simulink model "Control_Planta_LazoCerrado"  (R2023b)
settings: Solver=VariableStepAuto  StartTime=0.0  StopTime=15  FixedStep=0.00001  RelTol=1e-3
values from neighbouring files (symbols this model uses):
  A_corriente = [0 1; -wn_corriente^2 -2*zeta_corriente*wn_corriente]    [SensoresReales.m]
  A_inv = [0 1; -wn_inv^2 -2*zeta_inv*wn_inv]    [SensoresReales.m]
  A_temp = -1/tau_temp    (= -0.05)    [SensoresReales.m]
  A_tita = [0 1; -wn_tita^2 -2*zeta_tita*wn_tita]    [SensoresReales.m]
  B_corriente = [0; wn_corriente^2]    [SensoresReales.m]
  B_inv = [0; wn_inv^2]    [SensoresReales.m]
  B_temp = 1/tau_temp    (= 0.05)    [SensoresReales.m]
  B_tita = [0; wn_tita^2]    [SensoresReales.m]
  C_corriente = [1 0]    [SensoresReales.m]
  C_inv = [1 0]    [SensoresReales.m]
  C_temp = 1    [SensoresReales.m]
  C_tita = [1 0]    [SensoresReales.m]
  D_corriente = 0    [SensoresReales.m]
  D_inv = 0    [SensoresReales.m]
  D_temp = 0    [SensoresReales.m]
  D_tita = 0    [SensoresReales.m]
  id_consigna = 0.5    [RdLazoCorriente.m]
  ketita = double(sol.ketita_s)    [PIDPolosObsReducidoEst.m]    (also in PolosObsReducidoEst.m)
  kew = double(sol.kew_s)    [PIDPolosObsReducidoEst.m]    (also in PolosObsReducidoEst.m)
  kewint = double(sol.kewint_s)    [PIDPolosObsReducidoEst.m]    (also in PolosObsReducidoEst.m = 0)
  Ra_prima = Lq/Tau    [RaLazoControlCorriente.m]
  Rd_prima = Ld/Tau_d    [RdLazoCorriente.m]
  Tau = -1/Pi    (= 0.0002)    [RaLazoControlCorriente.m]
  Ts = 0.0001    [TustinPID.m]
  Vs_max = 48 * sqrt(2) / sqrt(3)    [SensoresReales.m]
undefined symbols (not defined in the file or in its folder): alfa, beq, Cts, den_PIDTZ, DiscIntNeverNeededParam, g, id0, io0, iq0, Ismax, Isnom, Jeq, KEeq, kl, KTeq, lambda_m, Ld, Lls, Lq, num_PIDTZ, Pp, r, Rs, Rts_amb, tita0, Tqnom, Ts0, Tsmax, Vflnom, Wlnom, wm0, Wmnom
libraries: simulink x11, simulink_extras x8, eeTransforms x4, SignalEditorBlockLib x3, dspsigops x1, spsabctoAlphaBetaZeroLib x1
settings Model: Creator=Julian  LastModifiedBy=Gustavo

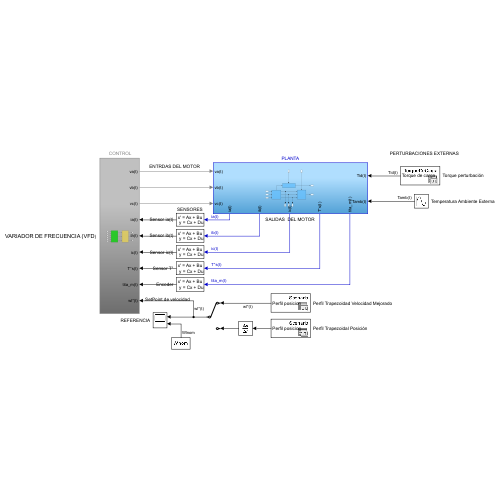
[thumbnail: Simulink's stored preview of the top-level diagram]
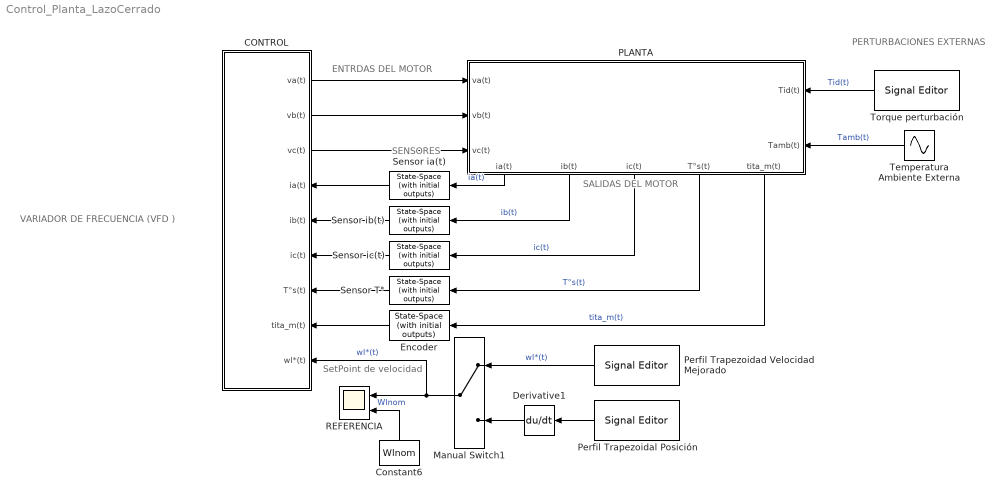
== system Control_Planta_LazoCerrado ==
  note: VARIADOR DE FRECUENCIA (VFD )
  note: SENSORES
  note: ENTRDAS DEL MOTOR
  note: PERTURBACIONES EXTERNAS
  note: SetPoint de velocidad
  note: SALIDAS DEL MOTOR
  " CONTROL" : Subsystem
      settings: PortSchema="{\"entries\":[{\"content\":{\"sides\":[{\"content\":{},\"type\":\"ConnectorPlacement.EquallySpacedRectSide\",\"uuid\":\"d9793d3b-98b9-44dc-9764-d251b8ee8eaa\"},{\"content\":{\"connectorIds\":[\"Out1\",\"Out2\",\"Out3\",\"In1\",\"In2\",\"In3\",\"In4\",\"In5\",\"In6\"],\"side\":\"RIGHT\"},\"type\":\"ConnectorPlacement.EquallySpacedRectSide\",\"uuid\":\"bdddef0b-c469-49f9-98ba-074ea9cbca1a\"},{\"content\":{\"side\":\"TOP\"},\"type\":\"ConnectorPlacement.EquallySpacedRectSide\",\"uuid\":\"8ca6b3a1-550b-497a-8309-d6b694c418e8\"}]},\"type\":\"ConnectorPlacement.EquallySpacedConnector\",\"uuid\":\"d8d4494b-c45d-4f5a-9083-73b1f67c784a\"}],\"packageUris\":[\"http://schema.mathworks.com/mf0/Connector/R2020b\"],\"version\":\"1.0\"}"
  Constant6 : Constant  Value=Wlnom
  Derivative1 : Derivative
  Encoder : simulink_extras/Additional Linear/State-Space (with initial outputs)  A=A_tita  B=B_tita  C=C_tita  D=D_tita  U0=0  Y0=0
  Manual Switch1 : ManualSwitch
  PLANTA : Subsystem
      settings: PortSchema="{\"entries\":[{\"content\":{\"sides\":[{\"content\":{\"connectorIds\":[\"In1\",\"In2\",\"In3\"]},\"type\":\"ConnectorPlacement.EquallySpacedRectSide\",\"uuid\":\"c9ff8e03-575d-49b6-9d53-263c6173ec7a\"},{\"content\":{\"connectorIds\":[\"In4\",\"In5\"],\"side\":\"RIGHT\"},\"type\":\"ConnectorPlacement.EquallySpacedRectSide\",\"uuid\":\"b812656a-111e-4032-91bd-eba1e3276cdf\"},{\"content\":{\"side\":\"TOP\"},\"type\":\"ConnectorPlacement.EquallySpacedRectSide\",\"uuid\":\"1a03caaa-7f6e-4ad3-ab54-ee47607f786a\"},{\"content\":{\"connectorIds\":[\"Out1\",\"Out2\",\"Out3\",\"Out4\",\"Out5\"],\"side\":\"BOTTOM\"},\"type\":\"ConnectorPlacement.EquallySpacedRectSide\",\"uuid\":\"9d23a867-d392-4f38-a76b-2655c4618fc4\"}]},\"type\":\"ConnectorPlacement.EquallySpacedConnector\",\"uuid\":\"9323b1ce-1fa4-461e-b8aa-3e94b35b1dab\"}],\"packageUris\":[\"http://schema.mathworks.com/mf0/Connector/R2020b\"],\"version\":\"1.0\"}"
  Perfil Trapezoidad Velocidad Mejorado : SignalEditorBlockLib/Signal Editor  FileName=PerfilTrapezoidalVelocidadMejorado.mat  ActiveScenario=Scenario  ActiveSignal=Perfil posicion  IsBus=off  OutputBusObjectStr=Bus: BusObject  SampleTime=0  ZeroCross=off  OutputAfterFinalValue=Setting to zero  Unit=inherit  PreserveSignalName=on  ApplySigPropsToAllScenarios=on  ApplySigPropsToAllSignals=off
  Perfil Trapezoidal Posición : SignalEditorBlockLib/Signal Editor  FileName=Perfil trapezoidal de posicion.mat  ActiveScenario=Scenario  ActiveSignal=Perfil posicion  IsBus=off  OutputBusObjectStr=Bus: BusObject  SampleTime=0  ZeroCross=off  OutputAfterFinalValue=Setting to zero  Unit=inherit  PreserveSignalName=on  ApplySigPropsToAllScenarios=on  ApplySigPropsToAllSignals=off
  REFERENCIA : Scope  NumInputPorts=2
  Sensor T° : simulink_extras/Additional Linear/State-Space (with initial outputs)  A=A_temp  B=B_temp  C=C_temp  D=D_temp  U0=40  Y0=40
  Sensor ia(t) : simulink_extras/Additional Linear/State-Space (with initial outputs)  A=A_corriente  B=B_corriente  C=C_corriente  D=D_corriente  U0=0  Y0=0
  Sensor ib(t) : simulink_extras/Additional Linear/State-Space (with initial outputs)  A=A_corriente  B=B_corriente  C=C_corriente  D=D_corriente  U0=0  Y0=0
  Sensor ic(t) : simulink_extras/Additional Linear/State-Space (with initial outputs)  A=A_corriente  B=B_corriente  C=C_corriente  D=D_corriente  U0=0  Y0=0
  Temperatura Ambiente Externa : Sin  Amplitude=27.5  Bias=12.5  Frequency=2*pi/15  Phase=pi/2  SampleTime=0
  Torque perturbación : SignalEditorBlockLib/Signal Editor  FileName=Torque de carga Tdl(t).mat  ActiveScenario=TorqueDeCarga  ActiveSignal=Torque de carga  IsBus=off  OutputBusObjectStr=Bus: BusObject  SampleTime=0  ZeroCross=off  OutputAfterFinalValue=Setting to zero  Unit=N*m  PreserveSignalName=on  ApplySigPropsToAllScenarios=on  ApplySigPropsToAllSignals=off
  wires:
  Torque perturbación/1 -> PLANTA/4(Tid(t))  "Tid(t)"
  PLANTA/5(tita_m(t)) -> Encoder/1  "tita_m(t)"
  PLANTA/1(ia(t)) -> Sensor ia(t)/1  "ia(t)"
  Manual Switch1/1 -> " CONTROL"/6(wl*(t)), REFERENCIA/1  "wl*(t)"
  Perfil Trapezoidad Velocidad Mejorado/1 -> Manual Switch1/1  "wl*(t)"
  Perfil Trapezoidal Posición/1 -> Derivative1/1
  Derivative1/1 -> Manual Switch1/2
  Constant6/1 -> REFERENCIA/2  "Wlnom"
  Temperatura Ambiente Externa/1 -> PLANTA/5(Tamb(t))  "Tamb(t)"
  PLANTA/4(T°s(t)) -> Sensor T°/1  "T°s(t)"
  PLANTA/2(ib(t)) -> Sensor ib(t)/1  "ib(t)"
  " CONTROL"/1(va(t)) -> PLANTA/1(va(t))
  " CONTROL"/2(vb(t)) -> PLANTA/2(vb(t))
  " CONTROL"/3(vc(t)) -> PLANTA/3(vc(t))
  Sensor ia(t)/1 -> " CONTROL"/1(ia(t))
  Sensor ib(t)/1 -> " CONTROL"/2(ib(t))
  Sensor ic(t)/1 -> " CONTROL"/3(ic(t))
  PLANTA/3(ic(t)) -> Sensor ic(t)/1  "ic(t)"
  Encoder/1 -> " CONTROL"/5(tita_m(t))
  Sensor T°/1 -> " CONTROL"/4(T°s(t))

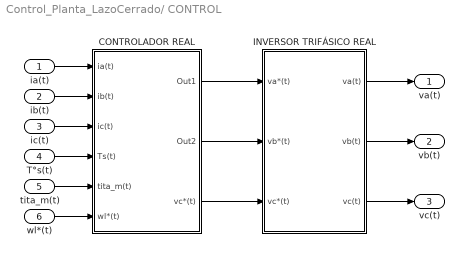
== system Control_Planta_LazoCerrado/ CONTROL ==
  ia(t) : Inport
  ib(t) : Inport  Port=2
  ic(t) : Inport  Port=3
  T°s(t) : Inport  Port=4
  tita_m(t) : Inport  Port=5
  wl*(t) : Inport  Port=6
  CONTROLADOR REAL : Subsystem
  INVERSOR TRIFÁSICO REAL : Subsystem
  va(t) : Outport
  vb(t) : Outport  Port=2
  vc(t) : Outport  Port=3
  wires:
  T°s(t)/1 -> CONTROLADOR REAL/4(Ts(t))
  CONTROLADOR REAL/2(Out2) -> INVERSOR TRIFÁSICO REAL/2(vb*(t))
  CONTROLADOR REAL/1(Out1) -> INVERSOR TRIFÁSICO REAL/1(va*(t))
  wl*(t)/1 -> CONTROLADOR REAL/6(wl*(t))
  INVERSOR TRIFÁSICO REAL/2(vb(t)) -> vb(t)/1
  ib(t)/1 -> CONTROLADOR REAL/2(ib(t))
  CONTROLADOR REAL/3(vc*(t)) -> INVERSOR TRIFÁSICO REAL/3(vc*(t))
  ia(t)/1 -> CONTROLADOR REAL/1(ia(t))
  ic(t)/1 -> CONTROLADOR REAL/3(ic(t))
  INVERSOR TRIFÁSICO REAL/1(va(t)) -> va(t)/1
  INVERSOR TRIFÁSICO REAL/3(vc(t)) -> vc(t)/1
  tita_m(t)/1 -> CONTROLADOR REAL/5(tita_m(t))

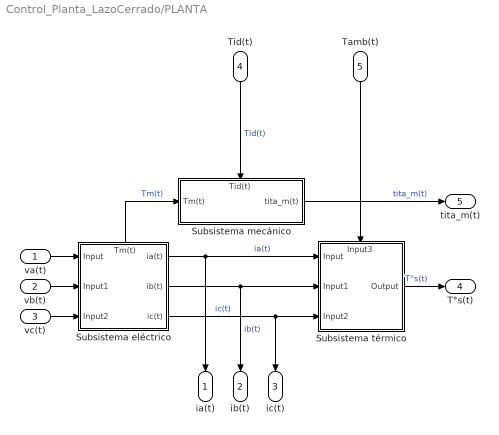
== system Control_Planta_LazoCerrado/PLANTA ==
  va(t) : Inport
  vb(t) : Inport  Port=2
  vc(t) : Inport  Port=3
  Tid(t) : Inport  Port=4
  Tamb(t) : Inport  Port=5
  Subsistema eléctrico : Subsystem
      settings: PortSchema="{\"entries\":[{\"content\":{\"sides\":[{\"content\":{\"connectorIds\":[\"In1\",\"In2\",\"In3\"]},\"type\":\"ConnectorPlacement.EquallySpacedRectSide\",\"uuid\":\"55314de5-b6ab-4161-b15d-819ac9b3d610\"},{\"content\":{\"connectorIds\":[\"Out1\",\"Out2\",\"Out3\"],\"side\":\"RIGHT\"},\"type\":\"ConnectorPlacement.EquallySpacedRectSide\",\"uuid\":\"6d89c228-26ff-4db5-b942-5bfef0be2fde\"},{\"content\":{\"connectorIds\":[\"Out4\"],\"side\":\"TOP\"},\"type\":\"ConnectorPlacement.EquallySpacedRectSide\",\"uuid\":\"a52f3ca3-a7f6-4886-b92b-9c9e6a107711\"}]},\"type\":\"ConnectorPlacement.EquallySpacedConnector\",\"uuid\":\"22991da4-d60d-4ddc-8bfe-b68e23663f11\"}],\"packageUris\":[\"http://schema.mathworks.com/mf0/Connector/R2020b\"],\"version\":\"1.0\"}"
  Subsistema mecánico : Subsystem
      settings: PortSchema="{\"entries\":[{\"content\":{\"sides\":[{\"content\":{\"connectorIds\":[\"In1\"]},\"type\":\"ConnectorPlacement.EquallySpacedRectSide\",\"uuid\":\"db0c31ff-fb9a-4cce-bd75-6b297d65744d\"},{\"content\":{\"connectorIds\":[\"Out1\"],\"side\":\"RIGHT\"},\"type\":\"ConnectorPlacement.EquallySpacedRectSide\",\"uuid\":\"ab44173d-bb84-4ea2-b7b7-ef15b1ff9d5e\"},{\"content\":{\"connectorIds\":[\"In2\"],\"side\":\"TOP\"},\"type\":\"ConnectorPlacement.EquallySpacedRectSide\",\"uuid\":\"a2ba5669-abba-4e87-b14b-37ec0d904023\"}]},\"type\":\"ConnectorPlacement.EquallySpacedConnector\",\"uuid\":\"7722c9ef-afaa-4930-9e2a-97c0dfb446ab\"}],\"packageUris\":[\"http://schema.mathworks.com/mf0/Connector/R2020b\"],\"version\":\"1.0\"}"
  Subsistema térmico : Subsystem
      settings: PortSchema="{\"entries\":[{\"content\":{\"sides\":[{\"content\":{\"connectorIds\":[\"In1\",\"In2\",\"In3\"]},\"type\":\"ConnectorPlacement.EquallySpacedRectSide\",\"uuid\":\"499bb5e3-da94-498d-be5e-1974ba0b4a58\"},{\"content\":{\"connectorIds\":[\"Out1\"],\"side\":\"RIGHT\"},\"type\":\"ConnectorPlacement.EquallySpacedRectSide\",\"uuid\":\"13ea5dea-e51e-4770-b579-88e3e6e50884\"},{\"content\":{\"connectorIds\":[\"In4\"],\"side\":\"TOP\"},\"type\":\"ConnectorPlacement.EquallySpacedRectSide\",\"uuid\":\"72517ed1-a98f-428e-86e2-c370e237c602\"}]},\"type\":\"ConnectorPlacement.EquallySpacedConnector\",\"uuid\":\"7e0eda24-12d6-49d0-ad1f-024c88e78140\"}],\"packageUris\":[\"http://schema.mathworks.com/mf0/Connector/R2020b\"],\"version\":\"1.0\"}"
  ia(t) : Outport
  ib(t) : Outport  Port=2
  ic(t) : Outport  Port=3
  T°s(t) : Outport  Port=4
  tita_m(t) : Outport  Port=5
  wires:
  Tamb(t)/1 -> Subsistema térmico/4(Input3)
  Subsistema eléctrico/3(ic(t)) -> Subsistema térmico/3(Input2), ic(t)/1  "ic(t)"
  Subsistema eléctrico/1(ia(t)) -> Subsistema térmico/1(Input), ia(t)/1  "ia(t)"
  Subsistema térmico/1(Output) -> T°s(t)/1  "T°s(t)"
  Subsistema eléctrico/4(Tm(t)) -> Subsistema mecánico/1(Tm(t))  "Tm(t)"
  Subsistema eléctrico/2(ib(t)) -> Subsistema térmico/2(Input1), ib(t)/1  "ib(t)"
  Subsistema mecánico/1(tita_m(t)) -> tita_m(t)/1  "tita_m(t)"
  va(t)/1 -> Subsistema eléctrico/1(Input)
  vb(t)/1 -> Subsistema eléctrico/2(Input1)
  Tid(t)/1 -> Subsistema mecánico/2(Tid(t))  "Tid(t)"
  vc(t)/1 -> Subsistema eléctrico/3(Input2)

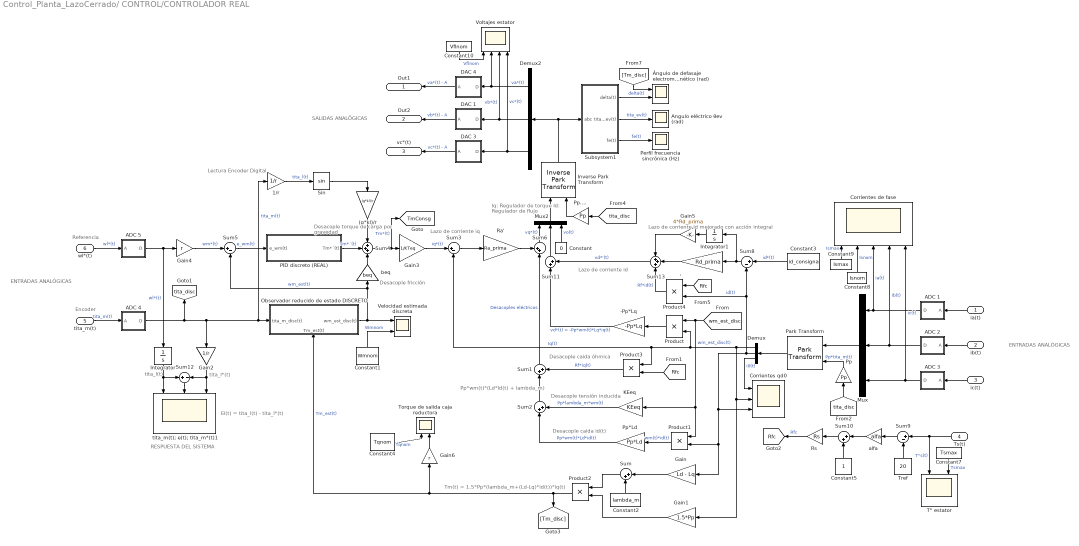
== system Control_Planta_LazoCerrado/ CONTROL/CONTROLADOR REAL ==
  note: Lazo de corriente id mejorado con acción integral
  note: Iq: Regulador de torque
      | Id: Regulador de flujo
  note: Lazo de corriente id
  note: ENTRADAS ANALÓGICAS
  note: SALIDAS ANALÖGICAS
  note: Desacople caida id(t)
  note: Encoder
  note: Desacople caida óhmica
  note: Desacople fricción
  note: Desacople tensión inducida
  note: Pp*wm(t)*(Ld*Id(t) + lambda_m)
  note: Lectura Encoder Digital
  note: Desacople torque
      | de carga por gravedad
  note: Tm(t) = 1.5*Pp*(lambda_m+(Ld-Lq)*id(t))*iq(t)
  note: ENTRADAS ANALÓGICAS
  note: Referencia
  note: Lazo de corriente iq
  note: tita_l*(t)
  note: RESPUESTA DEL SISTEMA
  note: El(t) = tita_l(t) - tita_l*(t)
  note: tita_l(t)
  ia(t) : Inport
  ib(t) : Inport  Port=2
  ic(t) : Inport  Port=3
  Ts(t) : Inport  Port=4
  tita_m(t) : Inport  Port=5
  wl*(t) : Inport  Port=6
  ' : Gain  Gain=Rd_prima
  (g*kl)/r : Gain  Gain=(g*kl)/r
  -Pp*Lq : Gain  Gain=-Pp*Lq
  1/r : Gain  Gain=1/r
  ADC 1 : Subsystem
  ADC 2 : Subsystem
  ADC 3 : Subsystem
  ADC 4 : Subsystem
  ADC 5 : Subsystem
  Angulo eléctrico θev (rad) : Scope
  Constant : Constant  Value=0
  Constant1 : Constant  Value=Wmnom
  Constant10 : Constant  Value=Vflnom
  Constant2 : Constant  Value=lambda_m
  Constant3 : Constant  Value=id_consigna
  Constant4 : Constant  Value=Tqnom
  Constant5 : Constant
  Constant7 : Constant  Value=Tsmax
  Constant8 : Constant  Value=Isnom
  Constant9 : Constant  Value=Ismax
  Corrientes de fase : Scope  NumInputPorts=5
  Corrientes qd0 : Scope  NumInputPorts=3
  DAC 1 : Subsystem
  DAC 3 : Subsystem
  DAC 4 : Subsystem
  Demux : Demux  Outputs=3
  Demux2 : Demux  Outputs=3
  Gain : Gain  Gain=Ld - Lq
  Gain1 : Gain  Gain=1.5*Pp
  Gain2 : Gain  Gain=1/r
  Gain3 : Gain  Gain=1/KTeq
  Gain4 : Gain  Gain=r
  Gain5 : Gain  Gain=4*Rd_prima
  Gain6 : Gain  Gain=r
  Integrator : Integrator
  Integrator1 : Integrator
  Inverse Park Transform : eeTransforms/Inverse Park Transform  AxisAlignment=Q-axis  PowerInvariant=off
      settings: LibrarySourceBlock=|
      | ee_sl_lib/Mathematical
      | Transforms/Inverse
      | Park Transform
  KEeq : Gain  Gain=KEeq
  Mux : Mux  Inputs=3
  Mux2 : Mux  Inputs=3
  Observador reducido de estado DISCRETO : Subsystem
      settings: PortSchema="{\"entries\":[{\"content\":{\"sides\":[{\"content\":{\"connectorIds\":[\"In1\"]},\"type\":\"ConnectorPlacement.EquallySpacedRectSide\",\"uuid\":\"14c71593-68f9-47eb-b449-943d4a083251\"},{\"content\":{\"connectorIds\":[\"Out1\"],\"side\":\"RIGHT\"},\"type\":\"ConnectorPlacement.EquallySpacedRectSide\",\"uuid\":\"16b08435-5727-4596-8f16-f9c2ce0b209d\"},{\"content\":{\"side\":\"TOP\"},\"type\":\"ConnectorPlacement.EquallySpacedRectSide\",\"uuid\":\"cb5316ed-c33b-4267-9a86-77fc386a7eee\"},{\"content\":{\"connectorIds\":[\"In2\"],\"side\":\"BOTTOM\"},\"type\":\"ConnectorPlacement.EquallySpacedRectSide\",\"uuid\":\"5f586da6-a83e-437c-ae41-e23b930b940a\"}]},\"type\":\"ConnectorPlacement.EquallySpacedConnector\",\"uuid\":\"0742f703-5bdc-4b50-9418-7ea0767d1226\"}],\"packageUris\":[\"http://schema.mathworks.com/mf0/Connector/R2020b\"],\"version\":\"1.0\"}"
  PID discreto (REAL) : Subsystem
  Park Transform : eeTransforms/Park Transform  AxisAlignment=Q-axis  PowerInvariant=off
      settings: LibrarySourceBlock=|
      | ee_sl_lib/Mathematical
      | Transforms/Park Transform
  Perfil frecuencia sincrónica (Hz) : Scope
  Pp : Gain  Gain=Pp
  Pp*Ld : Gain  Gain=Pp*Ld
  Pp.... : Gain  Gain=Pp
  Product{,1..4} (5 alike) : Product
  Ra' : Gain  Gain=Ra_prima
  Rs : Gain  Gain=Rs
  Sin : Trigonometry
  Subsystem1 : Subsystem
  Sum{,1..2,10..11} (5 alike) : Sum  Inputs=|++
  Sum12 : Sum  Inputs=+|-
  Sum13 : Sum  Inputs=+++
  Sum{3,5,8..9} (4 alike) : Sum  Inputs=|+-
  Sum4 : Sum  Inputs=+++
  Sum6 : Sum  Inputs=++|
  Torque de salida caja reductora : Scope  NumInputPorts=2
  Tref : Constant  Value=20
  T° estator : Scope  NumInputPorts=2
  Velocidad estimada discreta : Scope  NumInputPorts=2
  Voltajes estator : Scope  NumInputPorts=4
  alfa : Gain  Gain=alfa
  beq : Gain  Gain=beq
  tita_m(t); e(t); tita_m*(t)1 : Scope  NumInputPorts=3
  Ángulo de defasaje electromagnético (rad) : Scope  NumInputPorts=2
  Out1 : Outport
  Out2 : Outport  Port=2
  vc*(t) : Outport  Port=3
  tag scope: Rfc=global, TmConsg=global, tita_disc=global
  wires:
  Mux/1 -> Park Transform/1
  [tita_disc] -> Pp..../1
  Pp..../1 -> Inverse Park Transform/2
  Constant/1 -> Mux2/3  "vo(t)"
  Product3/1 -> Sum1/2  "Rf*iq(t)"
  [tita_disc] -> Pp/1
  Ra'/1 -> Sum6/1
  Inverse Park Transform/1 -> Subsystem1/1(abc), Demux2/1
  KEeq/1 -> Sum2/2  "Pp*lambda_m*wm(t)"
  Product1/1 -> Pp*Ld/1  "wm(t)*id(t)"
  Mux2/1 -> Inverse Park Transform/1
  Sum2/1 -> Sum1/1
  wl*(t)/1 -> ADC 5/1(A)  "wl*(t)"
  Pp*Ld/1 -> Sum2/1  "Pp*wm(t)*Ld*id(t)"
  Gain3/1 -> Sum3/1  "iq*(t)"
  Product/1 -> -Pp*Lq/1
  Park Transform/1 -> Demux/1
  Pp/1 -> Park Transform/2  "Pp*tita_m(t)"
  Sum6/1 -> Mux2/1  "vq*(t)"
  tita_m(t)/1 -> ADC 4/1(A)  "tita_m(t)"
  [Rfc] -> Product3/2
  Sum1/1 -> Sum6/2  "Desacoples eléctricos"
  Sum4/1 -> [TmConsg], Gain3/1  "Tm*(t)"
  beq/1 -> Sum4/3
  Observador reducido de estado DISCRETO/1(wm_est_disc(t)) -> Sum5/2, beq/1, Velocidad estimada discreta/1  "wm_est(t)"
  Demux/3 -> Corrientes qd0/1  "i0(t)"
  Demux/1 -> Product3/1, Sum3/2, Product/2, Gain1/1, Corrientes qd0/2  "Iq(t)"
  1/r/1 -> Sin/1  "tita_l(t)"
  Sin/1 -> (g*kl)/r/1
  (g*kl)/r/1 -> Sum4/1
  [wm_est_disc] -> Product1/1, KEeq/1, Product/1  "wm_est_disc(t)"
  Constant1/1 -> Velocidad estimada discreta/2  "Wmnom"
  ia(t)/1 -> ADC 1/1(A)
  ib(t)/1 -> ADC 2/1(A)
  ic(t)/1 -> ADC 3/1(A)
  ADC 1/1(D) -> Corrientes de fase/3, Mux/1  "ia(t)"
  Sum/1 -> Product2/1
  Constant2/1 -> Sum/2
  Gain1/1 -> Product2/2
  Gain/1 -> Sum/1
  DAC 4/1(A) -> Out1/1  "va*(t) - A"
  DAC 1/1(A) -> Out2/1  "vb*(t) - A"
  DAC 3/1(A) -> vc*(t)/1  "vc*(t) - A"
  Sum3/1 -> Ra'/1
  PID discreto (REAL)/1(Tm*´(t)) -> Sum4/2  "Tm*´(t)"
  Sum5/1 -> PID discreto (REAL)/1(e_wm(t))  "e_wm(t)"
  Subsystem1/2(tita_ev(t)) -> Angulo eléctrico θev (rad)/1  "tita_ev(t)"
  Subsystem1/1(delta(t)) -> Ángulo de defasaje electromagnético (rad)/2  "delta(t)"
  Subsystem1/3(fe(t)) -> Perfil frecuencia sincrónica (Hz)/1  "fe(t)"
  Sum9/1 -> alfa/1
  Sum10/1 -> Rs/1
  Rs/1 -> [Rfc]  "Rfc"
  [Rfc] -> Product4/1
  Product4/1 -> Sum13/3  "Rf*id(t)"
  Constant3/1 -> Sum8/1  "id*(t)"
  Sum8/1 -> Integrator1/1, '/1
  Demux/2 -> Sum8/2, Product4/2, Gain/1, Product1/2, Corrientes qd0/3  "id(t)"
  -Pp*Lq/1 -> Sum11/1  "vd*(t) = -Pp*wm(t)*Lq*iq(t)"
  Sum11/1 -> Mux2/2
  [Tm_disc] -> Ángulo de defasaje electromagnético (rad)/1
  Tref/1 -> Sum9/2
  Constant5/1 -> Sum10/2
  alfa/1 -> Sum10/1
  Demux2/3 -> DAC 3/1(D), Voltajes estator/4  "vc*(t)"
  Demux2/1 -> Voltajes estator/2, DAC 4/1(D)  "va*(t)"
  Demux2/2 -> DAC 1/1(D), Voltajes estator/3  "vb*(t)"
  Constant10/1 -> Voltajes estator/1  "Vflnom"
  Constant9/1 -> Corrientes de fase/1  "Ismax"
  ADC 3/1(D) -> Corrientes de fase/5, Mux/3  "ic(t)"
  ADC 2/1(D) -> Corrientes de fase/4, Mux/2  "ib(t)"
  Constant8/1 -> Corrientes de fase/2  "Isnom"
  Ts(t)/1 -> Sum9/1, T° estator/1  "T°s(t)"
  Constant7/1 -> T° estator/2  "Tsmax"
  ADC 4/1(D) -> Gain2/1, 1/r/1, Observador reducido de estado DISCRETO/1(tita_m_disc(t)), [tita_disc]  "tita_m(t)"
  ADC 5/1(D) -> Gain4/1, Integrator/1  "wl*(t)"
  Sum12/1 -> tita_m(t); e(t); tita_m*(t)1/2
  Gain4/1 -> Sum5/1  "wm*(t)"
  Gain2/1 -> Sum12/2, tita_m(t); e(t); tita_m*(t)1/3
  Integrator/1 -> tita_m(t); e(t); tita_m*(t)1/1, Sum12/1
  Sum13/1 -> Sum11/2  "vd*'(t)"
  Integrator1/1 -> Gain5/1
  Gain5/1 -> Sum13/1
  '/1 -> Sum13/2
  Product2/1 -> [Tm_disc], Gain6/1, Observador reducido de estado DISCRETO/2(Tm_est(t))  "Tm_est(t)"
  Gain6/1 -> Torque de salida caja reductora/2
  Constant4/1 -> Torque de salida caja reductora/1  "Tqnom"

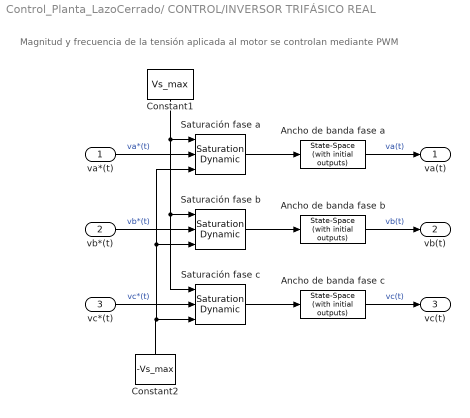
== system Control_Planta_LazoCerrado/ CONTROL/INVERSOR TRIFÁSICO REAL ==
  note: Magnitud y frecuencia de la tensión aplicada al motor se controlan mediante PWM
  va*(t) : Inport
  vb*(t) : Inport  Port=2
  vc*(t) : Inport  Port=3
  Ancho de banda fase a : simulink_extras/Additional Linear/State-Space (with initial outputs)  A=A_inv  B=B_inv  C=C_inv  D=D_inv  U0=0  Y0=0
  Ancho de banda fase b : simulink_extras/Additional Linear/State-Space (with initial outputs)  A=A_inv  B=B_inv  C=C_inv  D=D_inv  U0=0  Y0=0
  Ancho de banda fase c : simulink_extras/Additional Linear/State-Space (with initial outputs)  A=A_inv  B=B_inv  C=C_inv  D=D_inv  U0=0  Y0=0
  Constant1 : Constant  Value=Vs_max
  Constant2 : Constant  Value=-Vs_max
  Saturación fase a : simulink/Discontinuities/Saturation Dynamic  OutMin=[]  OutMax=[]  OutDataTypeStr=Inherit: Same as second input  OutDataType=fixdt(1, 16)  OutScaling=2^-10  DoSatur=off
  Saturación fase b : simulink/Discontinuities/Saturation Dynamic  OutMin=[]  OutMax=[]  OutDataTypeStr=Inherit: Same as second input  OutDataType=fixdt(1, 16)  OutScaling=2^-10  DoSatur=off
  Saturación fase c : simulink/Discontinuities/Saturation Dynamic  OutMin=[]  OutMax=[]  OutDataTypeStr=Inherit: Same as second input  OutDataType=fixdt(1, 16)  OutScaling=2^-10  DoSatur=off
  va(t) : Outport
  vb(t) : Outport  Port=2
  vc(t) : Outport  Port=3
  wires:
  Constant2/1 -> Saturación fase c/3, Saturación fase a/3, Saturación fase b/3
  va*(t)/1 -> Saturación fase a/2  "va*(t)"
  Saturación fase c/1 -> Ancho de banda fase c/1
  vc*(t)/1 -> Saturación fase c/2  "vc*(t)"
  vb*(t)/1 -> Saturación fase b/2  "vb*(t)"
  Saturación fase b/1 -> Ancho de banda fase b/1
  Saturación fase a/1 -> Ancho de banda fase a/1
  Constant1/1 -> Saturación fase c/1, Saturación fase b/1, Saturación fase a/1
  Ancho de banda fase b/1 -> vb(t)/1  "vb(t)"
  Ancho de banda fase a/1 -> va(t)/1  "va(t)"
  Ancho de banda fase c/1 -> vc(t)/1  "vc(t)"

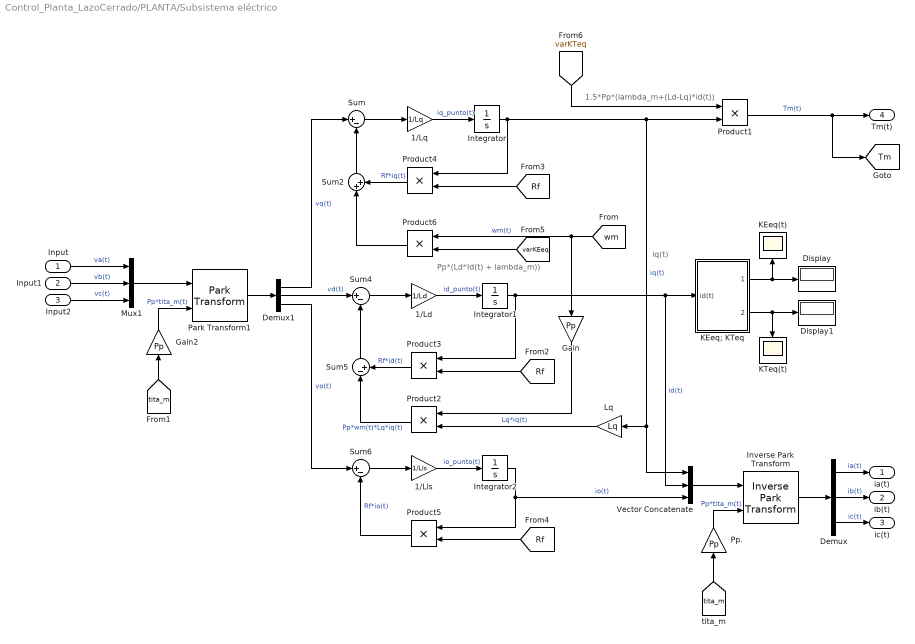
== system Control_Planta_LazoCerrado/PLANTA/Subsistema eléctrico ==
  note: 1.5*Pp*(lambda_m+(Ld-Lq)*id(t))
  note: iq(t)
  note: Pp*(Ld*Id(t) + lambda_m))
  Input : Inport
  Input1 : Inport  Port=2
  Input2 : Inport  Port=3
  1/Ld : Gain  Gain=1/Ld
  1/Lls : Gain  Gain=1/Lls
  1/Lq : Gain  Gain=1/Lq
  Demux : Demux  Outputs=3
  Demux1 : Demux  Outputs=3
  Display : Display
  Display1 : Display
  Gain : Gain  Gain=Pp
  Gain2 : Gain  Gain=Pp
  Integrator : Integrator  InitialCondition=iq0
  Integrator1 : Integrator  InitialCondition=id0
  Integrator2 : Integrator  InitialCondition=io0
  Inverse Park Transform : eeTransforms/Inverse Park Transform  AxisAlignment=Q-axis  PowerInvariant=off
      settings: LibrarySourceBlock=|
      | ee_sl_lib/Mathematical
      | Transforms/Inverse
      | Park Transform
  KEeq(t) : Scope
  KEeq; KTeq : Subsystem
  KTeq(t) : Scope
  Lq : Gain  Gain=Lq
  Mux1 : Mux  Inputs=3
  Park Transform1 : eeTransforms/Park Transform  AxisAlignment=Q-axis  PowerInvariant=off
      settings: LibrarySourceBlock=|
      | ee_sl_lib/Mathematical
      | Transforms/Park Transform
  Pp. : Gain  Gain=Pp
  Product{1..6} (6 alike) : Product
  Sum : Sum  Inputs=|+-
  Sum2 : Sum  Inputs=|++
  Sum4 : Sum  Inputs=|+-
  Sum5 : Sum  Inputs=|-+
  Sum6 : Sum  Inputs=|+-
  Vector Concatenate : Concatenate  NumInputs=3
  ia(t) : Outport
  ib(t) : Outport  Port=2
  ic(t) : Outport  Port=3
  Tm(t) : Outport  Port=4
  tag scope: Tm=global
  wires:
  Sum4/1 -> 1/Ld/1
  Demux1/1 -> Sum/1  "vq(t)"
  Integrator/1 -> Product4/1, Product1/2, Lq/1, Vector Concatenate/1  "iq(t)"
  Product4/1 -> Sum2/2  "Rf*iq(t)"
  Pp./1 -> Inverse Park Transform/2  "Pp*tita_m(t)"
  Lq/1 -> Product2/2  "Lq*iq(t)"
  Sum/1 -> 1/Lq/1
  Sum2/1 -> Sum/2
  Demux1/3 -> Sum6/1  "vo(t)"
  Vector Concatenate/1 -> Inverse Park Transform/1
  1/Ld/1 -> Integrator1/1  "id_punto(t)"
  Inverse Park Transform/1 -> Demux/1
  1/Lls/1 -> Integrator2/1  "io_punto(t)"
  Sum5/1 -> Sum4/2
  Demux/3 -> ic(t)/1  "ic(t)"
  Demux/1 -> ia(t)/1  "ia(t)"
  Product3/1 -> Sum5/2  "Rf*id(t)"
  Demux/2 -> ib(t)/1  "ib(t)"
  Integrator2/1 -> Product5/1, Vector Concatenate/3  "io(t)"
  [tita_m] -> Pp./1
  Demux1/2 -> Sum4/1  "vd(t)"
  Product6/1 -> Sum2/1
  Product5/1 -> Sum6/2  "Rf*io(t)"
  Product2/1 -> Sum5/1  "Pp*wm(t)*Lq*iq(t)"
  1/Lq/1 -> Integrator/1  "iq_punto(t)"
  Sum6/1 -> 1/Lls/1
  [wm] -> Product6/1, Gain/1  "wm(t)"
  Product1/1 -> Tm(t)/1, [Tm]  "Tm(t)"
  Input1/1 -> Mux1/2  "vb(t)"
  Gain2/1 -> Park Transform1/2  "Pp*tita_m(t)"
  Input2/1 -> Mux1/3  "vc(t)"
  Mux1/1 -> Park Transform1/1
  Input/1 -> Mux1/1  "va(t)"
  [tita_m] -> Gain2/1
  Park Transform1/1 -> Demux1/1
  [Rf] -> Product3/2
  [Rf] -> Product4/2
  [Rf] -> Product5/2
  Integrator1/1 -> Product3/1, KEeq; KTeq/1(id(t)), Vector Concatenate/2  "id(t)"
  [varKEeq] -> Product6/2
  Gain/1 -> Product2/1
  [varKTeq] -> Product1/1
  KEeq; KTeq/2(KTeq(t)) -> Display1/1, KTeq(t)/1
  KEeq; KTeq/1(KEeq(t)) -> KEeq(t)/1, Display/1

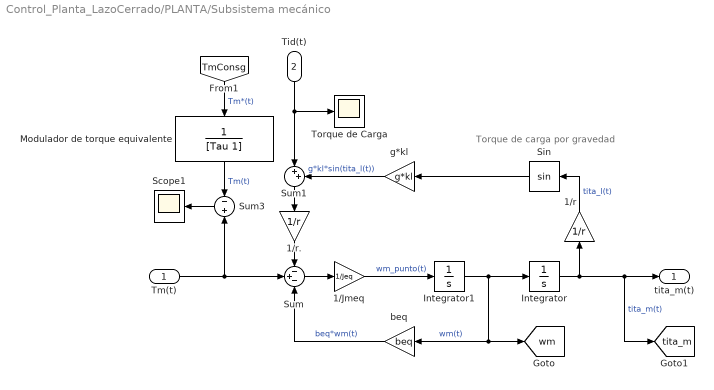
== system Control_Planta_LazoCerrado/PLANTA/Subsistema mecánico ==
  note: Torque de carga por gravedad
  Tm(t) : Inport
  Tid(t) : Inport  Port=2
  1/Jmeq : Gain  Gain=1/Jeq
  1/r : Gain  Gain=1/r
  1/r. : Gain  Gain=1/r
  Integrator : Integrator  InitialCondition=tita0
  Integrator1 : Integrator  InitialCondition=wm0
  Modulador de torque equivalente : TransferFcn  Denominator=[Tau 1]
  Scope1 : Scope
  Sin : Trigonometry
  Sum : Sum  Inputs=-+-
  Sum1 : Sum  Inputs=|++
  Sum3 : Sum  Inputs=-|+
  Torque de Carga : Scope
  beq : Gain  Gain=beq
  g*kl : Gain  Gain=g*kl
  tita_m(t) : Outport
  tag scope: tita_m=global, wm=global
  wires:
  Integrator/1 -> [tita_m], tita_m(t)/1, 1/r/1  "tita_m(t)"
  1/r./1 -> Sum/1
  Integrator1/1 -> beq/1, [wm], Integrator/1  "wm(t)"
  1/r/1 -> Sin/1  "tita_l(t)"
  Sin/1 -> g*kl/1
  Sum/1 -> 1/Jmeq/1
  1/Jmeq/1 -> Integrator1/1  "wm_punto(t)"
  beq/1 -> Sum/3  "beq*wm(t)"
  Tid(t)/1 -> Sum1/1, Torque de Carga/1
  Sum1/1 -> 1/r./1
  g*kl/1 -> Sum1/2  "g*kl*sin(tita_l(t))"
  Modulador de torque equivalente/1 -> Sum3/1  "Tm(t)"
  Tm(t)/1 -> Sum3/2, Sum/2
  Sum3/1 -> Scope1/1
  [TmConsg] -> Modulador de torque equivalente/1  "Tm*(t)"

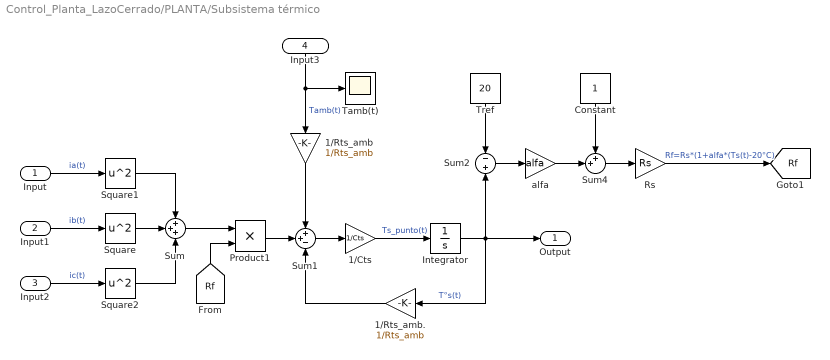
== system Control_Planta_LazoCerrado/PLANTA/Subsistema térmico ==
  Input : Inport
  Input1 : Inport  Port=2
  Input2 : Inport  Port=3
  Input3 : Inport  Port=4
  1/Cts : Gain  Gain=1/Cts
  1/Rts_amb : Gain  Gain=1/Rts_amb
  1/Rts_amb. : Gain  Gain=1/Rts_amb
  Constant : Constant
  Integrator : Integrator  InitialCondition=Ts0
  Product1 : Product
  Rs : Gain  Gain=Rs
  Square : Math  Operator=square
  Square1 : Math  Operator=square
  Square2 : Math  Operator=square
  Sum : Sum  Inputs=+++
  Sum1 : Sum  Inputs=++-
  Sum2 : Sum  Inputs=-+
  Sum4 : Sum  Inputs=++|
  Tamb(t) : Scope
  Tref : Constant  Value=20
  alfa : Gain  Gain=alfa
  Output : Outport
  tag scope: Rf=global
  wires:
  1/Rts_amb/1 -> Sum1/1
  Sum1/1 -> 1/Cts/1
  Product1/1 -> Sum1/2
  Sum/1 -> Product1/1
  Integrator/1 -> Sum2/2, Output/1, 1/Rts_amb./1  "T°s(t)"
  1/Cts/1 -> Integrator/1  "Ts_punto(t)"
  1/Rts_amb./1 -> Sum1/3
  Square/1 -> Sum/2
  Square1/1 -> Sum/1
  Square2/1 -> Sum/3
  Input/1 -> Square1/1  "ia(t)"
  Input1/1 -> Square/1  "ib(t)"
  Input2/1 -> Square2/1  "ic(t)"
  Sum2/1 -> alfa/1
  Constant/1 -> Sum4/1
  alfa/1 -> Sum4/2
  Rs/1 -> [Rf]  "Rf=Rs*(1+alfa*(Ts(t)-20°C)"
  [Rf] -> Product1/2
  Tref/1 -> Sum2/1
  Sum4/1 -> Rs/1
  Input3/1 -> 1/Rts_amb/1, Tamb(t)/1  "Tamb(t)"

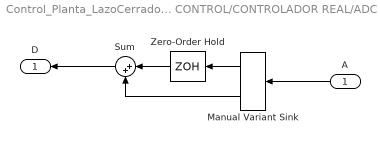
== system Control_Planta_LazoCerrado/ CONTROL/CONTROLADOR REAL/ADC 1 ==
  A : Inport
  Manual Variant Sink : simulink/Signal Routing/Manual Variant Sink  NumChoices=2  LabelModeActiveChoice=V_2
  Sum : Sum  Inputs=|++
  Zero-Order Hold : ZeroOrderHold  SampleTime=Ts
  D : Outport
  wires:
  Zero-Order Hold/1 -> Sum/1
  Sum/1 -> D/1
  Manual Variant Sink/2 -> Sum/2
  A/1 -> Manual Variant Sink/1
  Manual Variant Sink/1 -> Zero-Order Hold/1

== system Control_Planta_LazoCerrado/ CONTROL/CONTROLADOR REAL/ADC 2 ==
  A : Inport
  Manual Variant Sink : simulink/Signal Routing/Manual Variant Sink  NumChoices=2  LabelModeActiveChoice=V_2
  Sum : Sum  Inputs=|++
  Zero-Order Hold : ZeroOrderHold  SampleTime=Ts
  D : Outport
  wires:
  Manual Variant Sink/1 -> Zero-Order Hold/1
  A/1 -> Manual Variant Sink/1
  Manual Variant Sink/2 -> Sum/2
  Sum/1 -> D/1
  Zero-Order Hold/1 -> Sum/1

== system Control_Planta_LazoCerrado/ CONTROL/CONTROLADOR REAL/ADC 3 ==
  A : Inport
  Manual Variant Sink : simulink/Signal Routing/Manual Variant Sink  NumChoices=2  LabelModeActiveChoice=V_2
  Sum : Sum  Inputs=|++
  Zero-Order Hold : ZeroOrderHold  SampleTime=Ts
  D : Outport
  wires:
  Zero-Order Hold/1 -> Sum/1
  Sum/1 -> D/1
  Manual Variant Sink/2 -> Sum/2
  A/1 -> Manual Variant Sink/1
  Manual Variant Sink/1 -> Zero-Order Hold/1

== system Control_Planta_LazoCerrado/ CONTROL/CONTROLADOR REAL/ADC 4 ==
  A : Inport
  Manual Variant Sink : simulink/Signal Routing/Manual Variant Sink  NumChoices=2  LabelModeActiveChoice=V_2
  Sum : Sum  Inputs=|++
  Zero-Order Hold : ZeroOrderHold  SampleTime=Ts
  D : Outport
  wires:
  Manual Variant Sink/1 -> Zero-Order Hold/1
  A/1 -> Manual Variant Sink/1
  Manual Variant Sink/2 -> Sum/2
  Sum/1 -> D/1
  Zero-Order Hold/1 -> Sum/1

== system Control_Planta_LazoCerrado/ CONTROL/CONTROLADOR REAL/ADC 5 ==
  A : Inport
  Manual Variant Sink : simulink/Signal Routing/Manual Variant Sink  NumChoices=2  LabelModeActiveChoice=V_2
  Sum : Sum  Inputs=|++
  Zero-Order Hold : ZeroOrderHold  SampleTime=Ts
  D : Outport
  wires:
  Zero-Order Hold/1 -> Sum/1
  Sum/1 -> D/1
  Manual Variant Sink/2 -> Sum/2
  A/1 -> Manual Variant Sink/1
  Manual Variant Sink/1 -> Zero-Order Hold/1

== system Control_Planta_LazoCerrado/ CONTROL/CONTROLADOR REAL/DAC 1 ==
  D : Inport
  First Order Hold4 : FirstOrderHold  ErrorTolerance=inf  AllowContinuousInput=on
  Manual Variant Sink : simulink/Signal Routing/Manual Variant Sink  NumChoices=2  LabelModeActiveChoice=V_2
  Sum : Sum  Inputs=|++
  A : Outport
  wires:
  Manual Variant Sink/2 -> Sum/2
  Sum/1 -> A/1
  First Order Hold4/1 -> Sum/1
  D/1 -> Manual Variant Sink/1
  Manual Variant Sink/1 -> First Order Hold4/1

== system Control_Planta_LazoCerrado/ CONTROL/CONTROLADOR REAL/DAC 3 ==
  D : Inport
  First Order Hold4 : FirstOrderHold  ErrorTolerance=inf  AllowContinuousInput=on
  Manual Variant Sink : simulink/Signal Routing/Manual Variant Sink  NumChoices=2  LabelModeActiveChoice=V_2
  Sum : Sum  Inputs=|++
  A : Outport
  wires:
  Manual Variant Sink/1 -> First Order Hold4/1
  D/1 -> Manual Variant Sink/1
  First Order Hold4/1 -> Sum/1
  Sum/1 -> A/1
  Manual Variant Sink/2 -> Sum/2

== system Control_Planta_LazoCerrado/ CONTROL/CONTROLADOR REAL/DAC 4 ==
  D : Inport
  First Order Hold4 : FirstOrderHold  ErrorTolerance=inf  AllowContinuousInput=on
  Manual Variant Sink : simulink/Signal Routing/Manual Variant Sink  NumChoices=2  LabelModeActiveChoice=V_2
  Sum : Sum  Inputs=|++
  A : Outport
  wires:
  Manual Variant Sink/2 -> Sum/2
  Sum/1 -> A/1
  First Order Hold4/1 -> Sum/1
  D/1 -> Manual Variant Sink/1
  Manual Variant Sink/1 -> First Order Hold4/1

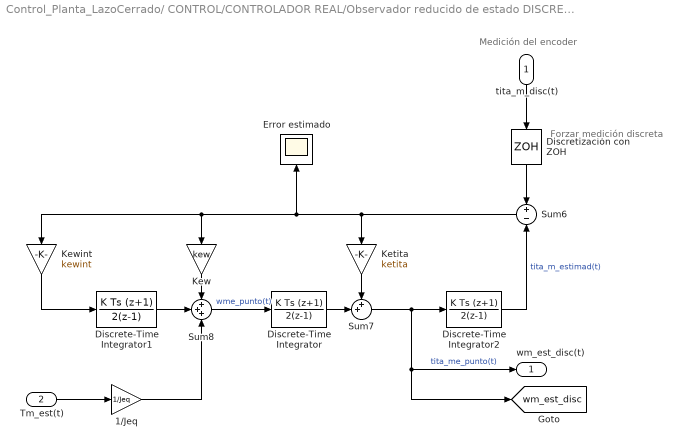
== system Control_Planta_LazoCerrado/ CONTROL/CONTROLADOR REAL/Observador reducido de estado DISCRETO ==
  note: Forzar medición discreta
  note: Medición del encoder
  tita_m_disc(t) : Inport
  Tm_est(t) : Inport  Port=2
  1/Jeq : Gain  Gain=1/Jeq
  Discrete-Time Integrator : DiscreteIntegrator  IntegratorMethod=Integration: Trapezoidal  SampleTime=Ts  ICPrevOutput=DiscIntNeverNeededParam  ICPrevScaledInput=DiscIntNeverNeededParam
  Discrete-Time Integrator1 : DiscreteIntegrator  IntegratorMethod=Integration: Trapezoidal  SampleTime=Ts  ICPrevOutput=DiscIntNeverNeededParam  ICPrevScaledInput=DiscIntNeverNeededParam
  Discrete-Time Integrator2 : DiscreteIntegrator  IntegratorMethod=Integration: Trapezoidal  SampleTime=Ts  ICPrevOutput=DiscIntNeverNeededParam  ICPrevScaledInput=DiscIntNeverNeededParam
  Discretización con ZOH : ZeroOrderHold  SampleTime=Ts
  Error estimado : Scope
  Ketita : Gain  Gain=ketita
  Kew : Gain  Gain=kew
  Kewint : Gain  Gain=kewint
  Sum6 : Sum  Inputs=+-
  Sum7 : Sum  Inputs=++|
  Sum8 : Sum  Inputs=+++
  wm_est_disc(t) : Outport
  tag scope: wm_est_disc=global
  wires:
  Sum7/1 -> [wm_est_disc], wm_est_disc(t)/1, Discrete-Time Integrator2/1  "tita_me_punto(t)"
  Sum6/1 -> Kewint/1, Kew/1, Error estimado/1, Ketita/1
  Discrete-Time Integrator2/1 -> Sum6/2  "tita_m_estimad(t)"
  Kew/1 -> Sum8/1
  Ketita/1 -> Sum7/1
  Sum8/1 -> Discrete-Time Integrator/1  "wme_punto(t)"
  tita_m_disc(t)/1 -> Discretización con ZOH/1
  1/Jeq/1 -> Sum8/3
  Discrete-Time Integrator/1 -> Sum7/2
  Discrete-Time Integrator1/1 -> Sum8/2
  Kewint/1 -> Discrete-Time Integrator1/1
  Discretización con ZOH/1 -> Sum6/1
  Tm_est(t)/1 -> 1/Jeq/1

== system Control_Planta_LazoCerrado/ CONTROL/CONTROLADOR REAL/PID discreto (REAL) ==
  e_wm(t) : Inport
  Función de transferencia PID discreto equivalente : DiscreteTransferFcn  Numerator=num_PIDTZ  Denominator=den_PIDTZ
  Señal discreta : Scope
  Zero-Order Hold : ZeroOrderHold  SampleTime=Ts
  Tm*´(t) : Outport
  wires:
  Función de transferencia PID discreto equivalente/1 -> Tm*´(t)/1, Señal discreta/1  "Tm*´(t)"
  e_wm(t)/1 -> Zero-Order Hold/1  "e_wm(t)"
  Zero-Order Hold/1 -> Función de transferencia PID discreto equivalente/1

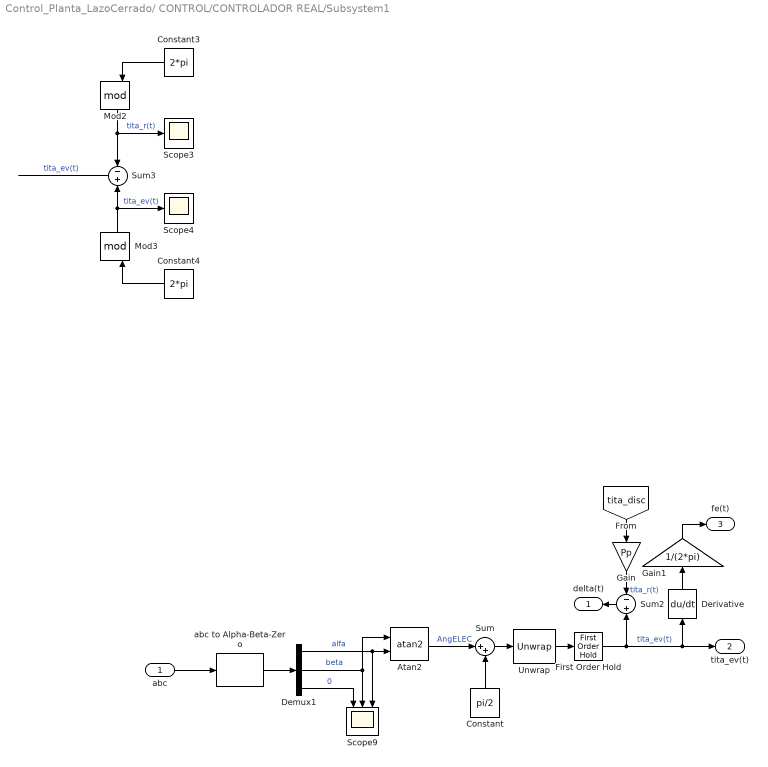
== system Control_Planta_LazoCerrado/ CONTROL/CONTROLADOR REAL/Subsystem1 ==
  abc : Inport
  Atan2 : Trigonometry  Operator=atan2
  Constant : Constant  Value=pi/2
  Constant3 : Constant  Value=2*pi
  Constant4 : Constant  Value=2*pi
  Demux1 : Demux  Outputs=3
  Derivative : Derivative
  First Order Hold : FirstOrderHold  ErrorTolerance=inf
  Gain : Gain  Gain=Pp
  Gain1 : Gain  Gain=1/(2*pi)
  Mod2 : Math  Operator=mod
  Mod3 : Math  Operator=mod
  Scope3 : Scope
  Scope4 : Scope
  Scope9 : Scope  NumInputPorts=3
  Sum : Sum  Inputs=|++
  Sum2 : Sum  Inputs=-|+
  Sum3 : Sum  Inputs=-|+
  Unwrap : dspsigops/Unwrap  tol=pi  InputProcessing=Columns as channels (frame based)  running=off
  abc to Alpha-Beta-Zero : spsabctoAlphaBetaZeroLib/abc to Alpha-Beta-Zero
  delta(t) : Outport
  tita_ev(t) : Outport  Port=2
  fe(t) : Outport  Port=3
  wires:
  Demux1/1 -> Scope9/3, Atan2/2  "alfa"
  abc to Alpha-Beta-Zero/1 -> Demux1/1
  Atan2/1 -> Sum/1  "AngELEC"
  Demux1/2 -> Scope9/2, Atan2/1  "beta"
  Constant/1 -> Sum/2
  Unwrap/1 -> First Order Hold/1
  Sum/1 -> Unwrap/1
  abc/1 -> abc to Alpha-Beta-Zero/1
  Demux1/3 -> Scope9/1  "0"
  First Order Hold/1 -> tita_ev(t)/1, Derivative/1, Sum2/2  "tita_ev(t)"
  Derivative/1 -> Gain1/1
  Gain1/1 -> fe(t)/1
  [tita_disc] -> Gain/1
  Gain/1 -> Sum2/1  "tita_r(t)"
  Sum2/1 -> delta(t)/1
  Constant4/1 -> Mod3/2
  ? -> Mod2/1  "tita_r(t)"
  Mod3/1 -> Scope4/1, Sum3/2  "tita_ev(t)"
  ? -> Mod3/1  "tita_ev(t)"
  Sum3/1 -> ?  "tita_ev(t)"
  Mod2/1 -> Sum3/1, Scope3/1  "tita_r(t)"
  Constant3/1 -> Mod2/2

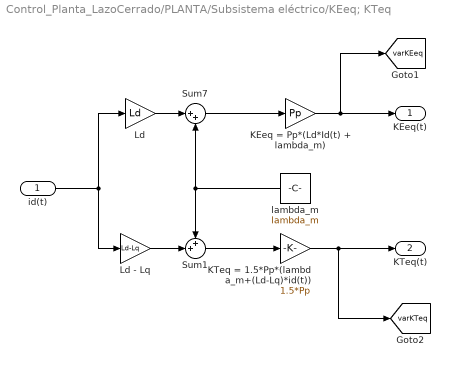
== system Control_Planta_LazoCerrado/PLANTA/Subsistema eléctrico/KEeq; KTeq ==
  id(t) : Inport
  "KEeq = Pp*(Ld*Id(t) + lambda_m) " : Gain  Gain=Pp
  "KTeq = 1.5*Pp*(lambda_m+(Ld-Lq)*id(t)) " : Gain  Gain=1.5*Pp
  Ld : Gain  Gain=Ld
  Ld - Lq : Gain  Gain=Ld-Lq
  Sum1 : Sum  Inputs=++|
  Sum7 : Sum  Inputs=|++
  lambda_m : Constant  Value=lambda_m
  KEeq(t) : Outport
  KTeq(t) : Outport  Port=2
  tag scope: varKEeq=global, varKTeq=global
  wires:
  Ld/1 -> Sum7/1
  Sum7/1 -> "KEeq = Pp*(Ld*Id(t) + lambda_m) "/1
  "KTeq = 1.5*Pp*(lambda_m+(Ld-Lq)*id(t)) "/1 -> KTeq(t)/1, [varKTeq]
  Sum1/1 -> "KTeq = 1.5*Pp*(lambda_m+(Ld-Lq)*id(t)) "/1
  id(t)/1 -> Ld/1, Ld - Lq/1
  Ld - Lq/1 -> Sum1/2
  lambda_m/1 -> Sum1/1, Sum7/2
  "KEeq = Pp*(Ld*Id(t) + lambda_m) "/1 -> [varKEeq], KEeq(t)/1
